simulink model "GaN_HalfBridge"  (R2016a)
settings: Solver=VariableStepAuto  StartTime=0.0  StopTime=1.4e-6  RelTol=1e-3
values from neighbouring files (symbols this model uses):
  Dbot = 49    [HalfBridge.m]    (also in HalfBridgeBottomConnectedLoad.m; HalfBridgeCapacitanceModelling.m)
  DelayBot = 50    [HalfBridge.m]    (also in HalfBridgeBottomConnectedLoad.m; HalfBridgeCapacitanceModelling.m)
  DelayTop = 0    [HalfBridge.m]    (also in HalfBridgeBottomConnectedLoad.m; HalfBridgeCapacitanceModelling.m)
  Dtop = 49    [HalfBridge.m]    (also in HalfBridgeBottomConnectedLoad.m; HalfBridgeCapacitanceModelling.m)
  fsw = 1e6    (= 1000000)    [ChannelAndDSTrajectories.m]    (also in GanModel_Nonsegmented.m = 100000; HalfBridge.m; HalfBridgeBottomConnectedLoad.m; HalfBridgeCapacitanceModelling.m)
  Rd = 3.6*0.95*0.82*18.2*0.25/295    (= 0.0432543050847)    [AnalyticalModel.m]    (also in GanModel_Nonsegmented.m = 0.1; HalfBridge.m = 0.025; HalfBridgeBottomConnectedLoad.m = 2.5e-05; HalfBridgeCapacitanceModelling.m = 2.5e-05)
  Rg = 1    [GanModel_Nonsegmented.m]    (also in HalfBridge.m; HalfBridgeBottomConnectedLoad.m = 1.5; HalfBridgeCapacitanceModelling.m = 1.5)
  Rload = 10    [GanModel_Nonsegmented.m]    (also in HalfBridge.m; HalfBridgeBottomConnectedLoad.m; HalfBridgeCapacitanceModelling.m = 5)
  Roff = 2    [HalfBridge.m]    (also in HalfBridgeBottomConnectedLoad.m; HalfBridgeCapacitanceModelling.m)
  Ron = 12    [HalfBridge.m]    (also in HalfBridgeBottomConnectedLoad.m; HalfBridgeCapacitanceModelling.m)
  Rs = 3.6*0.238*0.82/295    (= 0.00238161355932)    [AnalyticalModel.m]    (also in GanModel_Nonsegmented.m = 0.1; HalfBridge.m = 0.025; HalfBridgeBottomConnectedLoad.m = 2.5e-05; HalfBridgeCapacitanceModelling.m = 2.5e-05)
libraries: elec_lib x30, fl_lib x10, nesl_utility x10
settings Model: Creator=ugurm  LastModifiedBy=ugurm

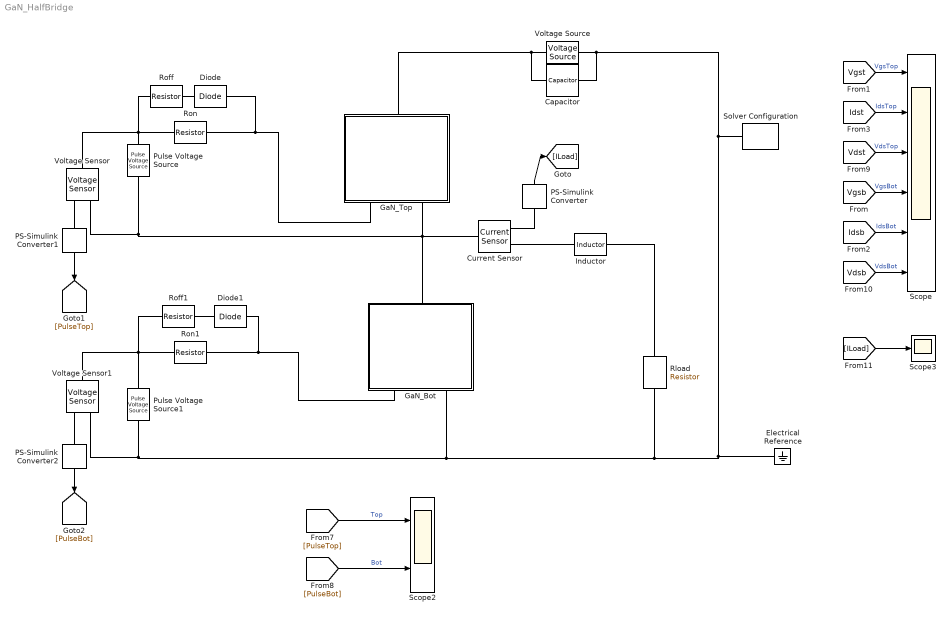
== system GaN_HalfBridge ==
  Capacitor : elec_lib/Passive Devices/Capacitor  enable_table=0  c=1e-3 F  Cvec=[ 1e-5 1e-6 ] F  Vvec=[ 0 10 ] V  CV_table_symmetry=1  C_tol=5  enable_C_tol=0  tol_distribution=1  nSigma=4  r=1e-6 Ohm  g=0 1/Ohm  initV=0 V  enable_operating_limits=0  operating_limit_action=2  max_working_voltage_range=[ -25 25 ] V  power_rating=1 W  enable_faults=0  fault_action=1  Cscale_faulted=100  R_faulted=0.001 Ohm  G_faulted=0 1/Ohm  tau_fault=0.001 s  enable_temporal_fault=0  t_fault=1 s  enable_behavioral_fault=0  max_permissible_voltage_range=[ -100 100 ] V  t_fail_on_voltage=1 s
  Current Sensor : fl_lib/Electrical/Electrical Sensors/Current Sensor
  Diode : elec_lib/Semiconductor Devices/Diode  ModelType=1  Vf=0.6 V  Ron=0.3 Ohm  Goff=1e-8 S  Rz=0.3 Ohm  Vz=50 V  C_PWL=5 pF  prmExp=1  I12=[ 0.0137 0.545 ] A  V12=[ 0.6 0.7 ] V  I1=0.0137 A  V1=0.6 V  RS=0.01 Ohm  IS=1e-12 A  Tmeas=25 degC  ec=1  BV=Inf V  C_param=1  CJ0=5 pF  VJ=1 V  Mgrad=0.5  Vvec=[ 0.1 10 100 ] V  Cvec=[ 3.5 1 0.4 ] pF  FC=0.5  Q_param=1  Irrm=-7.15 A  iF=4 A  didt=-750 A/us  trr=115 ns  TT=50 ns  tau=100 ns  T_param=1  IS_T2=1.25e-7 A  I1_T2=0.245 A  V1_T2=0.5 V  Tmeas2=125 degC  EG_param=1  EG=1.11 eV  XTI_param=1  XTI=3  dBVdT=0 V/K  Tdevice=25 degC  Rth=[ 0 10 ] K/W  thermal_mass_parameterization=1  thermal_mass=[ 0 1 ] J/K  thermal_time_constant=[ 0 10 ] s  thermal_mass_initial_temperatures=[ 25 25 ] degC
  Diode1 : elec_lib/Semiconductor Devices/Diode  ModelType=1  Vf=0.6 V  Ron=0.3 Ohm  Goff=1e-8 S  Rz=0.3 Ohm  Vz=50 V  C_PWL=5 pF  prmExp=1  I12=[ 0.0137 0.545 ] A  V12=[ 0.6 0.7 ] V  I1=0.0137 A  V1=0.6 V  RS=0.01 Ohm  IS=1e-12 A  Tmeas=25 degC  ec=1  BV=Inf V  C_param=1  CJ0=5 pF  VJ=1 V  Mgrad=0.5  Vvec=[ 0.1 10 100 ] V  Cvec=[ 3.5 1 0.4 ] pF  FC=0.5  Q_param=1  Irrm=-7.15 A  iF=4 A  didt=-750 A/us  trr=115 ns  TT=50 ns  tau=100 ns  T_param=1  IS_T2=1.25e-7 A  I1_T2=0.245 A  V1_T2=0.5 V  Tmeas2=125 degC  EG_param=1  EG=1.11 eV  XTI_param=1  XTI=3  dBVdT=0 V/K  Tdevice=25 degC  Rth=[ 0 10 ] K/W  thermal_mass_parameterization=1  thermal_mass=[ 0 1 ] J/K  thermal_time_constant=[ 0 10 ] s  thermal_mass_initial_temperatures=[ 25 25 ] degC
  Electrical Reference : fl_lib/Electrical/Electrical Elements/Electrical Reference
  GaN_Bot : Subsystem
  GaN_Top : Subsystem
  Inductor : elec_lib/Passive Devices/Inductor  l=Lload H  L_tol=20  enable_L_tol=0  tol_distribution=1  nSigma=4  r=0 Ohm  g=1e-9 1/Ohm  initI=0 A  enable_operating_limits=0  operating_limit_action=2  max_working_current=1 A  power_rating=1 W  enable_faults=0  fault_action=1  lambdaPercent=50  k_faulted=0.9999 Ohm  turnsShort=0  openCct=0  groundShort=0  groundShortG=0 1/Ohm  tau_fault=0.001 s  enable_temporal_fault=0  t_fault=1 s  enable_behavioral_fault=0  max_permissible_voltage=100 V  n_fail_on_voltage=1  max_permissible_current=1 A  t_fail_on_current=1 s
  PS-Simulink Converter : nesl_utility/PS-Simulink Converter  PhysicalDomain=network_engine_domain  SubClassName=ps_output  LeftPortType=input  RightPortType=output  PseudoPeriodic=off  Frequencies=[]  Unit=1  AffineConversion=off
  PS-Simulink Converter1 : nesl_utility/PS-Simulink Converter  PhysicalDomain=network_engine_domain  SubClassName=ps_output  LeftPortType=input  RightPortType=output  PseudoPeriodic=off  Frequencies=[]  Unit=1  AffineConversion=off
  PS-Simulink Converter2 : nesl_utility/PS-Simulink Converter  PhysicalDomain=network_engine_domain  SubClassName=ps_output  LeftPortType=input  RightPortType=output  PseudoPeriodic=off  Frequencies=[]  Unit=1  AffineConversion=off
  Pulse Voltage Source : elec_lib/Additional Components/SPICE-Compatible Components/Sources/Pulse Voltage Source  V1=-3 V  V2=PulseAmplitude V  TD=DelayTop/(100*fsw) s  TR=1e-9 s  TF=1e-9 s  PW=Dtop/(100*fsw) s  PER=1/fsw s
  Pulse Voltage Source1 : elec_lib/Additional Components/SPICE-Compatible Components/Sources/Pulse Voltage Source  V1=-3 V  V2=PulseAmplitude V  TD=DelayBot/(100*fsw) s  TR=1e-9 s  TF=1e-9 s  PW=Dbot/(100*fsw) s  PER=1/fsw s
  Rload : elec_lib/Passive Devices/Resistor  R=Rload Ohm  R_tol=5  enable_R_tol=0  tol_distribution=1  nSigma=4  enable_operating_limits=0  operating_limit_action=2  max_working_voltage=100 V  power_rating=1 W  enable_faults=0  fault_action=1  R_faulted=Inf Ohm  enable_temporal_fault=0  t_fault=1 s  enable_behavioral_fault=0  max_permissible_current=1 A  t_fail_on_current=1 s  noise_mode=0  sample_time=0.001 s  repeatability=1  auto_seed=3812810898  user_seed=0  Tdevice=25 degC  alpha=0.00393 1/K  Tmeas=25 degC  thermal_mass=100 J/K  initial_temperature=25 degC  power_derating_T1=70 degC  power_derating_T2=155 degC  operating_temperature_range_vec=[ -50 150 ] degC
  Roff : elec_lib/Passive Devices/Resistor  R=Roff Ohm  R_tol=5  enable_R_tol=0  tol_distribution=1  nSigma=4  enable_operating_limits=0  operating_limit_action=2  max_working_voltage=100 V  power_rating=1 W  enable_faults=0  fault_action=1  R_faulted=Inf Ohm  enable_temporal_fault=0  t_fault=1 s  enable_behavioral_fault=0  max_permissible_current=1 A  t_fail_on_current=1 s  noise_mode=0  sample_time=0.001 s  repeatability=1  auto_seed=935450722  user_seed=0  Tdevice=25 degC  alpha=0.00393 1/K  Tmeas=25 degC  thermal_mass=100 J/K  initial_temperature=25 degC  power_derating_T1=70 degC  power_derating_T2=155 degC  operating_temperature_range_vec=[ -50 150 ] degC
  Roff1 : elec_lib/Passive Devices/Resistor  R=Roff Ohm  R_tol=5  enable_R_tol=0  tol_distribution=1  nSigma=4  enable_operating_limits=0  operating_limit_action=2  max_working_voltage=100 V  power_rating=1 W  enable_faults=0  fault_action=1  R_faulted=Inf Ohm  enable_temporal_fault=0  t_fault=1 s  enable_behavioral_fault=0  max_permissible_current=1 A  t_fail_on_current=1 s  noise_mode=0  sample_time=0.001 s  repeatability=1  auto_seed=1550577895  user_seed=0  Tdevice=25 degC  alpha=0.00393 1/K  Tmeas=25 degC  thermal_mass=100 J/K  initial_temperature=25 degC  power_derating_T1=70 degC  power_derating_T2=155 degC  operating_temperature_range_vec=[ -50 150 ] degC
  Ron : elec_lib/Passive Devices/Resistor  R=Ron Ohm  R_tol=5  enable_R_tol=0  tol_distribution=1  nSigma=4  enable_operating_limits=0  operating_limit_action=2  max_working_voltage=100 V  power_rating=1 W  enable_faults=0  fault_action=1  R_faulted=Inf Ohm  enable_temporal_fault=0  t_fault=1 s  enable_behavioral_fault=0  max_permissible_current=1 A  t_fail_on_current=1 s  noise_mode=0  sample_time=0.001 s  repeatability=1  auto_seed=782289965  user_seed=0  Tdevice=25 degC  alpha=0.00393 1/K  Tmeas=25 degC  thermal_mass=100 J/K  initial_temperature=25 degC  power_derating_T1=70 degC  power_derating_T2=155 degC  operating_temperature_range_vec=[ -50 150 ] degC
  Ron1 : elec_lib/Passive Devices/Resistor  R=Ron Ohm  R_tol=5  enable_R_tol=0  tol_distribution=1  nSigma=4  enable_operating_limits=0  operating_limit_action=2  max_working_voltage=100 V  power_rating=1 W  enable_faults=0  fault_action=1  R_faulted=Inf Ohm  enable_temporal_fault=0  t_fault=1 s  enable_behavioral_fault=0  max_permissible_current=1 A  t_fail_on_current=1 s  noise_mode=0  sample_time=0.001 s  repeatability=1  auto_seed=2664075559  user_seed=0  Tdevice=25 degC  alpha=0.00393 1/K  Tmeas=25 degC  thermal_mass=100 J/K  initial_temperature=25 degC  power_derating_T1=70 degC  power_derating_T2=155 degC  operating_temperature_range_vec=[ -50 150 ] degC
  Scope : Scope  NumInputPorts=6
  Scope2 : Scope  NumInputPorts=2
  Scope3 : Scope
  Solver Configuration : nesl_utility/Solver Configuration  PhysicalDomain=network_engine_domain  SubClassName=solver  LeftPortType=input  RightPortType=generic  Accelerate=off  Tones=[]  Harmonics=[]  SimulateNoise=off  Profile=off  UseLocalSampling=off  EnableSwitchedLinearOptims=on  FrequencyDomain=off  UseCCode=off  RelTol=0.001  AbsTol=1e-06  MinStep=1e-09  ToWorkspace=off  RevertToSquareIcSolve=off  NumHomotopyIterations=100  PhasorMode=off  PhasorModeNumHarmonics=1  OverrideAbsTol=off  DoDC=off  ResidualTolerance=1e-09  UseLocalSolver=on  LocalSolverChoice=NE_BACKWARD_EULER_ADVANCER  LocalSolverSampleTime=SampleTime  DoFixedCost=on  MaxNonlinIter=3  MaxModeIter=2  LinearAlgebra=Sparse  DelaysMemoryBudget=1024  AutomaticFiltering=on  FilteringTimeConstant=0.001
  Voltage Sensor : fl_lib/Electrical/Electrical Sensors/Voltage Sensor
  Voltage Sensor1 : fl_lib/Electrical/Electrical Sensors/Voltage Sensor
  Voltage Source : elec_lib/Sources/Voltage Source  dc_voltage=Vdc V  ac_voltage=0 V  ac_shift=0 deg  ac_frequency=60 Hz  noise_mode=0  PSD=0 V^2/Hz  sample_time=0.001 s  repeatability=1  auto_seed=79941259  user_seed=0
  wires:
  PS-Simulink Converter/1 -> [ILoad]
  PS-Simulink Converter1/1 -> [PulseTop]
  PS-Simulink Converter2/1 -> [PulseBot]
  [PulseTop] -> Scope2/1  "Top"
  [PulseBot] -> Scope2/2  "Bot"
  [Vgsb] -> Scope/4  "VgsBot"
  [Idsb] -> Scope/5  "IdsBot"
  [Idst] -> Scope/2  "IdsTop"
  [Vgst] -> Scope/1  "VgsTop"
  [Vdst] -> Scope/3  "VdsTop"
  [Vdsb] -> Scope/6  "VdsBot"
  [ILoad] -> Scope3/1
  connections:
  Roff/RConn1 -- Ron/RConn1 -- Voltage Sensor/LConn1 -- Pulse Voltage Source/LConn1
  Diode/LConn1 -- Ron/LConn1 -- GaN_Top/LConn1
  Roff/LConn1 -- Diode/RConn1
  Voltage Source/LConn1 -- Capacitor/LConn1 -- GaN_Top/RConn1
  GaN_Top/LConn2 -- GaN_Bot/RConn1 -- Current Sensor/LConn1 -- Voltage Sensor/RConn2 -- Pulse Voltage Source/RConn1
  Pulse Voltage Source1/LConn1 -- Voltage Sensor1/LConn1 -- Ron1/RConn1 -- Roff1/RConn1
  Diode1/LConn1 -- GaN_Bot/LConn1 -- Ron1/LConn1
  Roff1/LConn1 -- Diode1/RConn1
  GaN_Bot/LConn2 -- Capacitor/RConn1 -- Voltage Source/RConn1 -- Solver Configuration/RConn1 -- Electrical Reference/LConn1 -- Rload/RConn1 -- Voltage Sensor1/RConn2 -- Pulse Voltage Source1/RConn1
  Inductor/RConn1 -- Rload/LConn1
  Current Sensor/RConn2 -- Inductor/LConn1
  PS-Simulink Converter/LConn1 -- Current Sensor/RConn1
  PS-Simulink Converter1/LConn1 -- Voltage Sensor/RConn1
  PS-Simulink Converter2/LConn1 -- Voltage Sensor1/RConn1

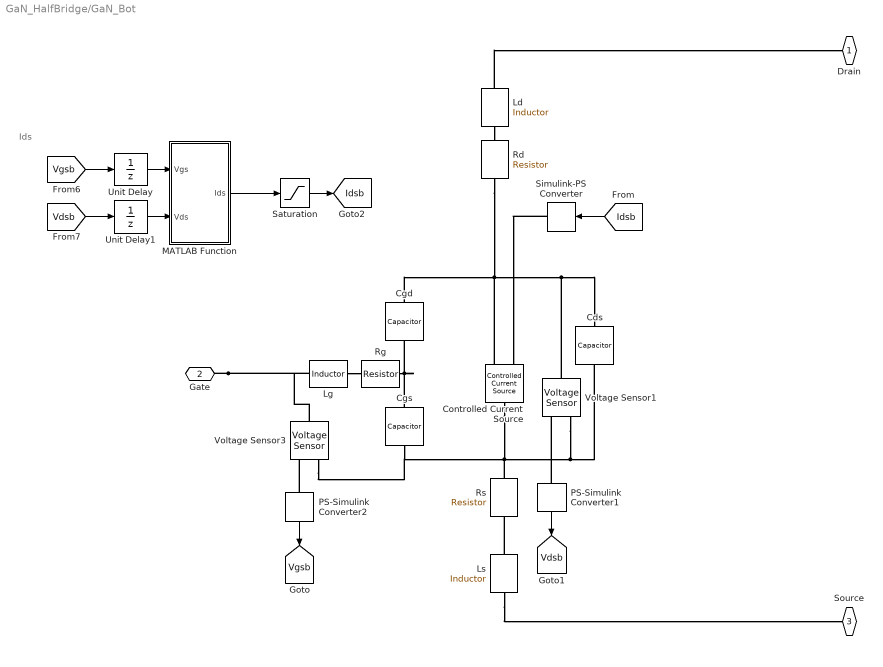
== system GaN_HalfBridge/GaN_Bot ==
  note: Ids
  Cds : elec_lib/Passive Devices/Capacitor  enable_table=0  c=Cds F  Cvec=[ 1e-5 1e-6 ] F  Vvec=[ 0 10 ] V  CV_table_symmetry=1  C_tol=5  enable_C_tol=0  tol_distribution=1  nSigma=4  r=1e-6 Ohm  g=0 1/Ohm  initV=0 V  enable_operating_limits=0  operating_limit_action=2  max_working_voltage_range=[ -25 25 ] V  power_rating=1 W  enable_faults=0  fault_action=1  Cscale_faulted=100  R_faulted=0.001 Ohm  G_faulted=0 1/Ohm  tau_fault=0.001 s  enable_temporal_fault=0  t_fault=1 s  enable_behavioral_fault=0  max_permissible_voltage_range=[ -100 100 ] V  t_fail_on_voltage=1 s
  Cgd : elec_lib/Passive Devices/Capacitor  enable_table=0  c=Cgd F  Cvec=[ 1e-5 1e-6 ] F  Vvec=[ 0 10 ] V  CV_table_symmetry=1  C_tol=5  enable_C_tol=0  tol_distribution=1  nSigma=4  r=1e-6 Ohm  g=0 1/Ohm  initV=0 V  enable_operating_limits=0  operating_limit_action=2  max_working_voltage_range=[ -25 25 ] V  power_rating=1 W  enable_faults=0  fault_action=1  Cscale_faulted=100  R_faulted=0.001 Ohm  G_faulted=0 1/Ohm  tau_fault=0.001 s  enable_temporal_fault=0  t_fault=1 s  enable_behavioral_fault=0  max_permissible_voltage_range=[ -100 100 ] V  t_fail_on_voltage=1 s
  Cgs : elec_lib/Passive Devices/Capacitor  enable_table=0  c=Cgs F  Cvec=[ 1e-5 1e-6 ] F  Vvec=[ 0 10 ] V  CV_table_symmetry=1  C_tol=5  enable_C_tol=0  tol_distribution=1  nSigma=4  r=1e-6 Ohm  g=0 1/Ohm  initV=0 V  enable_operating_limits=0  operating_limit_action=2  max_working_voltage_range=[ -25 25 ] V  power_rating=1 W  enable_faults=0  fault_action=1  Cscale_faulted=100  R_faulted=0.001 Ohm  G_faulted=0 1/Ohm  tau_fault=0.001 s  enable_temporal_fault=0  t_fault=1 s  enable_behavioral_fault=0  max_permissible_voltage_range=[ -100 100 ] V  t_fail_on_voltage=1 s
  Controlled Current Source : fl_lib/Electrical/Electrical Sources/Controlled Current Source
  Ld : elec_lib/Passive Devices/Inductor  l=Ld H  L_tol=5  enable_L_tol=0  tol_distribution=1  nSigma=4  r=0 Ohm  g=1e-9 1/Ohm  initI=0 A  enable_operating_limits=0  operating_limit_action=2  max_working_current=1 A  power_rating=1 W  enable_faults=0  fault_action=1  lambdaPercent=50  k_faulted=0.9999 Ohm  turnsShort=0  openCct=0  groundShort=0  groundShortG=0 1/Ohm  tau_fault=0.001 s  enable_temporal_fault=0  t_fault=1 s  enable_behavioral_fault=0  max_permissible_voltage=100 V  n_fail_on_voltage=1  max_permissible_current=1 A  t_fail_on_current=1 s
  Lg : elec_lib/Passive Devices/Inductor  l=Lg H  L_tol=5  enable_L_tol=0  tol_distribution=1  nSigma=4  r=0 Ohm  g=1e-9 1/Ohm  initI=0 A  enable_operating_limits=0  operating_limit_action=2  max_working_current=1 A  power_rating=1 W  enable_faults=0  fault_action=1  lambdaPercent=50  k_faulted=0.9999 Ohm  turnsShort=0  openCct=0  groundShort=0  groundShortG=0 1/Ohm  tau_fault=0.001 s  enable_temporal_fault=0  t_fault=1 s  enable_behavioral_fault=0  max_permissible_voltage=100 V  n_fail_on_voltage=1  max_permissible_current=1 A  t_fail_on_current=1 s
  Ls : elec_lib/Passive Devices/Inductor  l=Ls H  L_tol=5  enable_L_tol=0  tol_distribution=1  nSigma=4  r=0 Ohm  g=1e-9 1/Ohm  initI=0 A  enable_operating_limits=0  operating_limit_action=2  max_working_current=1 A  power_rating=1 W  enable_faults=0  fault_action=1  lambdaPercent=50  k_faulted=0.9999 Ohm  turnsShort=0  openCct=0  groundShort=0  groundShortG=0 1/Ohm  tau_fault=0.001 s  enable_temporal_fault=0  t_fault=1 s  enable_behavioral_fault=0  max_permissible_voltage=100 V  n_fail_on_voltage=1  max_permissible_current=1 A  t_fail_on_current=1 s
  MATLAB Function : MATLAB Function  TreatAsAtomicUnit=on
  PS-Simulink Converter1 : nesl_utility/PS-Simulink Converter  PhysicalDomain=network_engine_domain  SubClassName=ps_output  LeftPortType=input  RightPortType=output  PseudoPeriodic=off  Frequencies=[]  Unit=1  AffineConversion=off
  PS-Simulink Converter2 : nesl_utility/PS-Simulink Converter  PhysicalDomain=network_engine_domain  SubClassName=ps_output  LeftPortType=input  RightPortType=output  PseudoPeriodic=off  Frequencies=[]  Unit=1  AffineConversion=off
  Rd : elec_lib/Passive Devices/Resistor  R=Rd Ohm  R_tol=5  enable_R_tol=0  tol_distribution=1  nSigma=4  enable_operating_limits=0  operating_limit_action=2  max_working_voltage=100 V  power_rating=1 W  enable_faults=0  fault_action=1  R_faulted=Inf Ohm  enable_temporal_fault=0  t_fault=1 s  enable_behavioral_fault=0  max_permissible_current=1 A  t_fail_on_current=1 s  noise_mode=0  sample_time=0.001 s  repeatability=1  auto_seed=2865259871  user_seed=0  Tdevice=25 degC  alpha=0.00393 1/K  Tmeas=25 degC  thermal_mass=100 J/K  initial_temperature=25 degC  power_derating_T1=70 degC  power_derating_T2=155 degC  operating_temperature_range_vec=[ -50 150 ] degC
  Rg : elec_lib/Passive Devices/Resistor  R=Rg Ohm  R_tol=5  enable_R_tol=0  tol_distribution=1  nSigma=4  enable_operating_limits=0  operating_limit_action=2  max_working_voltage=100 V  power_rating=1 W  enable_faults=0  fault_action=1  R_faulted=Inf Ohm  enable_temporal_fault=0  t_fault=1 s  enable_behavioral_fault=0  max_permissible_current=1 A  t_fail_on_current=1 s  noise_mode=0  sample_time=0.001 s  repeatability=1  auto_seed=2518738966  user_seed=0  Tdevice=25 degC  alpha=0.00393 1/K  Tmeas=25 degC  thermal_mass=100 J/K  initial_temperature=25 degC  power_derating_T1=70 degC  power_derating_T2=155 degC  operating_temperature_range_vec=[ -50 150 ] degC
  Rs : elec_lib/Passive Devices/Resistor  R=Rs Ohm  R_tol=5  enable_R_tol=0  tol_distribution=1  nSigma=4  enable_operating_limits=0  operating_limit_action=2  max_working_voltage=100 V  power_rating=1 W  enable_faults=0  fault_action=1  R_faulted=Inf Ohm  enable_temporal_fault=0  t_fault=1 s  enable_behavioral_fault=0  max_permissible_current=1 A  t_fail_on_current=1 s  noise_mode=0  sample_time=0.001 s  repeatability=1  auto_seed=2899585749  user_seed=0  Tdevice=25 degC  alpha=0.00393 1/K  Tmeas=25 degC  thermal_mass=100 J/K  initial_temperature=25 degC  power_derating_T1=70 degC  power_derating_T2=155 degC  operating_temperature_range_vec=[ -50 150 ] degC
  Saturation : Saturate  UpperLimit=100  LowerLimit=-100
  Simulink-PS Converter : nesl_utility/Simulink-PS Converter  PhysicalDomain=network_engine_domain  SubClassName=ps_input  LeftPortType=input  RightPortType=output  PseudoPeriodic=off  Frequencies=[]  NoiseDistribution=none  NoiseParameters=[]  Unit=1  AffineConversion=off  InputFiltering=off  SimscapeFilterOrder=1  InputFilterTimeConstant=0.001  UdotUserProvided=1
  Unit Delay : UnitDelay  SampleTime=-1
  Unit Delay1 : UnitDelay  SampleTime=-1
  Voltage Sensor1 : fl_lib/Electrical/Electrical Sensors/Voltage Sensor
  Voltage Sensor3 : fl_lib/Electrical/Electrical Sensors/Voltage Sensor
  Drain : PMIOPort  Port=1  Side=Right
  Gate : PMIOPort  Port=2  Side=Left
  Source : PMIOPort  Port=3  Side=Left
  tag scope: Idsb=global, Vdsb=global, Vgsb=global
  wires:
  PS-Simulink Converter2/1 -> [Vgsb]
  Unit Delay1/1 -> MATLAB Function/2(Vds)
  Unit Delay/1 -> MATLAB Function/1(Vgs)
  MATLAB Function/1(Ids) -> Saturation/1
  [Vgsb] -> Unit Delay/1
  [Vdsb] -> Unit Delay1/1
  PS-Simulink Converter1/1 -> [Vdsb]
  Saturation/1 -> [Idsb]
  [Idsb] -> Simulink-PS Converter/1
  connections:
  Ld/LConn1 -- Drain/RConn1
  Ls/RConn1 -- Source/RConn1
  PS-Simulink Converter2/LConn1 -- Voltage Sensor3/RConn1
  Gate/RConn1 -- Lg/LConn1 -- Voltage Sensor3/LConn1
  Simulink-PS Converter/RConn1 -- Controlled Current Source/RConn1
  Ld/RConn1 -- Rd/LConn1
  Ls/LConn1 -- Rs/RConn1
  PS-Simulink Converter1/LConn1 -- Voltage Sensor1/RConn1
  Lg/RConn1 -- Rg/RConn1
  Cgs/RConn1 -- Voltage Sensor3/RConn2 -- Controlled Current Source/LConn1 -- Rs/LConn1 -- Voltage Sensor1/RConn2 -- Cds/RConn1
  Cgs/LConn1 -- Cgd/RConn1 -- Rg/LConn1
  Cgd/LConn1 -- Cds/LConn1 -- Voltage Sensor1/LConn1 -- Controlled Current Source/RConn2 -- Rd/RConn1

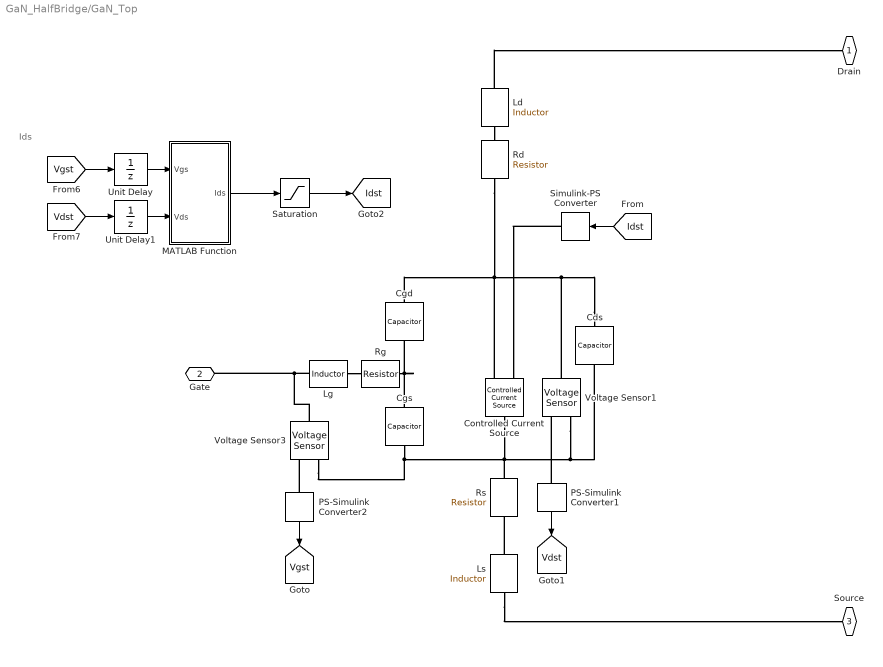
== system GaN_HalfBridge/GaN_Top ==
  note: Ids
  Cds : elec_lib/Passive Devices/Capacitor  enable_table=0  c=Cds F  Cvec=[ 1e-5 1e-6 ] F  Vvec=[ 0 10 ] V  CV_table_symmetry=1  C_tol=5  enable_C_tol=0  tol_distribution=1  nSigma=4  r=1e-6 Ohm  g=0 1/Ohm  initV=0 V  enable_operating_limits=0  operating_limit_action=2  max_working_voltage_range=[ -25 25 ] V  power_rating=1 W  enable_faults=0  fault_action=1  Cscale_faulted=100  R_faulted=0.001 Ohm  G_faulted=0 1/Ohm  tau_fault=0.001 s  enable_temporal_fault=0  t_fault=1 s  enable_behavioral_fault=0  max_permissible_voltage_range=[ -100 100 ] V  t_fail_on_voltage=1 s
  Cgd : elec_lib/Passive Devices/Capacitor  enable_table=0  c=Cgd F  Cvec=[ 1e-5 1e-6 ] F  Vvec=[ 0 10 ] V  CV_table_symmetry=1  C_tol=5  enable_C_tol=0  tol_distribution=1  nSigma=4  r=1e-6 Ohm  g=0 1/Ohm  initV=0 V  enable_operating_limits=0  operating_limit_action=2  max_working_voltage_range=[ -25 25 ] V  power_rating=1 W  enable_faults=0  fault_action=1  Cscale_faulted=100  R_faulted=0.001 Ohm  G_faulted=0 1/Ohm  tau_fault=0.001 s  enable_temporal_fault=0  t_fault=1 s  enable_behavioral_fault=0  max_permissible_voltage_range=[ -100 100 ] V  t_fail_on_voltage=1 s
  Cgs : elec_lib/Passive Devices/Capacitor  enable_table=0  c=Cgs F  Cvec=[ 1e-5 1e-6 ] F  Vvec=[ 0 10 ] V  CV_table_symmetry=1  C_tol=5  enable_C_tol=0  tol_distribution=1  nSigma=4  r=1e-6 Ohm  g=0 1/Ohm  initV=0 V  enable_operating_limits=0  operating_limit_action=2  max_working_voltage_range=[ -25 25 ] V  power_rating=1 W  enable_faults=0  fault_action=1  Cscale_faulted=100  R_faulted=0.001 Ohm  G_faulted=0 1/Ohm  tau_fault=0.001 s  enable_temporal_fault=0  t_fault=1 s  enable_behavioral_fault=0  max_permissible_voltage_range=[ -100 100 ] V  t_fail_on_voltage=1 s
  Controlled Current Source : fl_lib/Electrical/Electrical Sources/Controlled Current Source
  Ld : elec_lib/Passive Devices/Inductor  l=Ld H  L_tol=5  enable_L_tol=0  tol_distribution=1  nSigma=4  r=0 Ohm  g=1e-9 1/Ohm  initI=0 A  enable_operating_limits=0  operating_limit_action=2  max_working_current=1 A  power_rating=1 W  enable_faults=0  fault_action=1  lambdaPercent=50  k_faulted=0.9999 Ohm  turnsShort=0  openCct=0  groundShort=0  groundShortG=0 1/Ohm  tau_fault=0.001 s  enable_temporal_fault=0  t_fault=1 s  enable_behavioral_fault=0  max_permissible_voltage=100 V  n_fail_on_voltage=1  max_permissible_current=1 A  t_fail_on_current=1 s
  Lg : elec_lib/Passive Devices/Inductor  l=Lg H  L_tol=5  enable_L_tol=0  tol_distribution=1  nSigma=4  r=0 Ohm  g=1e-9 1/Ohm  initI=0 A  enable_operating_limits=0  operating_limit_action=2  max_working_current=1 A  power_rating=1 W  enable_faults=0  fault_action=1  lambdaPercent=50  k_faulted=0.9999 Ohm  turnsShort=0  openCct=0  groundShort=0  groundShortG=0 1/Ohm  tau_fault=0.001 s  enable_temporal_fault=0  t_fault=1 s  enable_behavioral_fault=0  max_permissible_voltage=100 V  n_fail_on_voltage=1  max_permissible_current=1 A  t_fail_on_current=1 s
  Ls : elec_lib/Passive Devices/Inductor  l=Ls H  L_tol=5  enable_L_tol=0  tol_distribution=1  nSigma=4  r=0 Ohm  g=1e-9 1/Ohm  initI=0 A  enable_operating_limits=0  operating_limit_action=2  max_working_current=1 A  power_rating=1 W  enable_faults=0  fault_action=1  lambdaPercent=50  k_faulted=0.9999 Ohm  turnsShort=0  openCct=0  groundShort=0  groundShortG=0 1/Ohm  tau_fault=0.001 s  enable_temporal_fault=0  t_fault=1 s  enable_behavioral_fault=0  max_permissible_voltage=100 V  n_fail_on_voltage=1  max_permissible_current=1 A  t_fail_on_current=1 s
  MATLAB Function : MATLAB Function  TreatAsAtomicUnit=on
  PS-Simulink Converter1 : nesl_utility/PS-Simulink Converter  PhysicalDomain=network_engine_domain  SubClassName=ps_output  LeftPortType=input  RightPortType=output  PseudoPeriodic=off  Frequencies=[]  Unit=1  AffineConversion=off
  PS-Simulink Converter2 : nesl_utility/PS-Simulink Converter  PhysicalDomain=network_engine_domain  SubClassName=ps_output  LeftPortType=input  RightPortType=output  PseudoPeriodic=off  Frequencies=[]  Unit=1  AffineConversion=off
  Rd : elec_lib/Passive Devices/Resistor  R=Rd Ohm  R_tol=5  enable_R_tol=0  tol_distribution=1  nSigma=4  enable_operating_limits=0  operating_limit_action=2  max_working_voltage=100 V  power_rating=1 W  enable_faults=0  fault_action=1  R_faulted=Inf Ohm  enable_temporal_fault=0  t_fault=1 s  enable_behavioral_fault=0  max_permissible_current=1 A  t_fail_on_current=1 s  noise_mode=0  sample_time=0.001 s  repeatability=1  auto_seed=3861196639  user_seed=0  Tdevice=25 degC  alpha=0.00393 1/K  Tmeas=25 degC  thermal_mass=100 J/K  initial_temperature=25 degC  power_derating_T1=70 degC  power_derating_T2=155 degC  operating_temperature_range_vec=[ -50 150 ] degC
  Rg : elec_lib/Passive Devices/Resistor  R=Rg Ohm  R_tol=5  enable_R_tol=0  tol_distribution=1  nSigma=4  enable_operating_limits=0  operating_limit_action=2  max_working_voltage=100 V  power_rating=1 W  enable_faults=0  fault_action=1  R_faulted=Inf Ohm  enable_temporal_fault=0  t_fault=1 s  enable_behavioral_fault=0  max_permissible_current=1 A  t_fail_on_current=1 s  noise_mode=0  sample_time=0.001 s  repeatability=1  auto_seed=2688381633  user_seed=0  Tdevice=25 degC  alpha=0.00393 1/K  Tmeas=25 degC  thermal_mass=100 J/K  initial_temperature=25 degC  power_derating_T1=70 degC  power_derating_T2=155 degC  operating_temperature_range_vec=[ -50 150 ] degC
  Rs : elec_lib/Passive Devices/Resistor  R=Rs Ohm  R_tol=5  enable_R_tol=0  tol_distribution=1  nSigma=4  enable_operating_limits=0  operating_limit_action=2  max_working_voltage=100 V  power_rating=1 W  enable_faults=0  fault_action=1  R_faulted=Inf Ohm  enable_temporal_fault=0  t_fault=1 s  enable_behavioral_fault=0  max_permissible_current=1 A  t_fail_on_current=1 s  noise_mode=0  sample_time=0.001 s  repeatability=1  auto_seed=179614949  user_seed=0  Tdevice=25 degC  alpha=0.00393 1/K  Tmeas=25 degC  thermal_mass=100 J/K  initial_temperature=25 degC  power_derating_T1=70 degC  power_derating_T2=155 degC  operating_temperature_range_vec=[ -50 150 ] degC
  Saturation : Saturate  UpperLimit=100  LowerLimit=-100
  Simulink-PS Converter : nesl_utility/Simulink-PS Converter  PhysicalDomain=network_engine_domain  SubClassName=ps_input  LeftPortType=input  RightPortType=output  PseudoPeriodic=off  Frequencies=[]  NoiseDistribution=none  NoiseParameters=[]  Unit=1  AffineConversion=off  InputFiltering=off  SimscapeFilterOrder=1  InputFilterTimeConstant=0.001  UdotUserProvided=1
  Unit Delay : UnitDelay  SampleTime=-1
  Unit Delay1 : UnitDelay  SampleTime=-1
  Voltage Sensor1 : fl_lib/Electrical/Electrical Sensors/Voltage Sensor
  Voltage Sensor3 : fl_lib/Electrical/Electrical Sensors/Voltage Sensor
  Drain : PMIOPort  Port=1  Side=Right
  Gate : PMIOPort  Port=2  Side=Left
  Source : PMIOPort  Port=3  Side=Left
  tag scope: Idst=global, Vdst=global, Vgst=global
  wires:
  PS-Simulink Converter1/1 -> [Vdst]
  [Vdst] -> Unit Delay1/1
  [Vgst] -> Unit Delay/1
  MATLAB Function/1(Ids) -> Saturation/1
  Unit Delay/1 -> MATLAB Function/1(Vgs)
  Unit Delay1/1 -> MATLAB Function/2(Vds)
  PS-Simulink Converter2/1 -> [Vgst]
  Saturation/1 -> [Idst]
  [Idst] -> Simulink-PS Converter/1
  connections:
  Cds/LConn1 -- Voltage Sensor1/LConn1 -- Cgd/LConn1 -- Rd/RConn1 -- Controlled Current Source/RConn2
  Cgd/RConn1 -- Cgs/LConn1 -- Rg/LConn1
  Voltage Sensor1/RConn2 -- Voltage Sensor3/RConn2 -- Cgs/RConn1 -- Rs/LConn1 -- Controlled Current Source/LConn1 -- Cds/RConn1
  Lg/RConn1 -- Rg/RConn1
  PS-Simulink Converter1/LConn1 -- Voltage Sensor1/RConn1
  Ls/LConn1 -- Rs/RConn1
  Ld/RConn1 -- Rd/LConn1
  Simulink-PS Converter/RConn1 -- Controlled Current Source/RConn1
  Lg/LConn1 -- Gate/RConn1 -- Voltage Sensor3/LConn1
  PS-Simulink Converter2/LConn1 -- Voltage Sensor3/RConn1
  Ls/RConn1 -- Source/RConn1
  Ld/LConn1 -- Drain/RConn1

== matlab function GaN_HalfBridge/GaN_Bot/MATLAB Function ==
  data: Vgs input; Ids output; Vds input
function Ids = fcn(Vgs,Vds)
%#codegen
K1 = 0.283;
b1 = 2.035;
c1 = 0.124;
d1 = 1.159;
e1 = -0.204;
m1 = 30.972;
n1 = -4.48;
K2 = 7.114;
b2 = 2.054;
c2 = 0.153;
Vgd = Vgs - Vds;
if Vds == 0
    Vds = 0.001;
end
if Vds>0
    Ids = K1*log(1+exp((Vgs-b1)/c1))*((m1+n1*Vgs)*Vds)/(1+(d1+e1*Vgs)*Vds);
else

    Ids = -K2*log(1+exp((Vgd-b2)/c2))*(-Vds/(1-Vds));
end

== matlab function GaN_HalfBridge/GaN_Top/MATLAB Function ==
  data: Vgs input; Ids output; Vds input
function Ids = fcn(Vgs,Vds)
%#codegen
K1 = 0.283;
b1 = 2.035;
c1 = 0.124;
d1 = 1.159;
e1 = -0.204;
m1 = 30.972;
n1 = -4.48;
K2 = 7.114;
b2 = 2.054;
c2 = 0.153;
Vgd = Vgs - Vds;
if Vds == 0
    Vds = 0.001;
end
if Vds>0
    Ids = K1*log(1+exp((Vgs-b1)/c1))*((m1+n1*Vgs)*Vds)/(1+(d1+e1*Vgs)*Vds);
else

    Ids = -K2*log(1+exp((Vgd-b2)/c2))*(-Vds/(1-Vds));
end
